simulink model "Ex1s"  (R2025a)
settings: Solver=VariableStepAuto  StartTime=0.0  StopTime=10.0  RelTol=1e-3

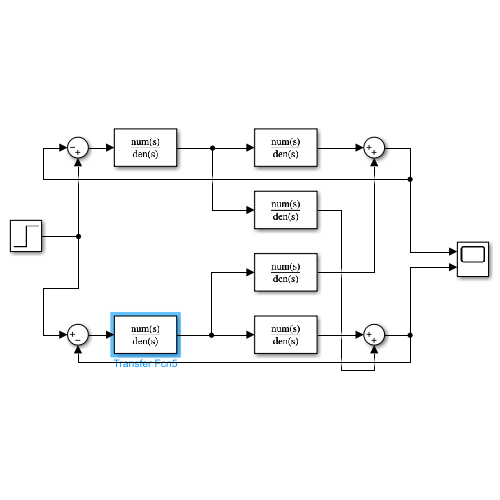
[thumbnail: Simulink's stored preview of the top-level diagram]
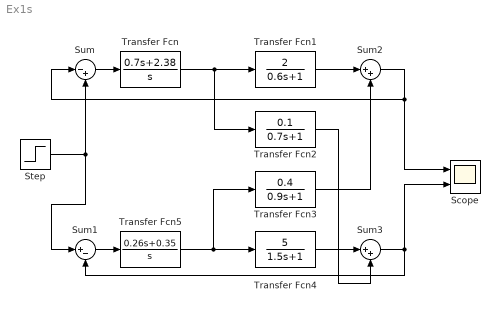
== system Ex1s ==
  Scope : Scope  NumInputPorts=2
      settings: ActiveDisplayYMinimum=-0.092364806170674857  ActiveDisplayYMaximum=0.83128325553607385
  Step : Step  SampleTime=0
  Sum : Sum  Inputs=|-+
  Sum1 : Sum  Inputs=|+-
  Sum2 : Sum  Inputs=|++
  Sum3 : Sum  Inputs=|++
  Transfer Fcn : TransferFcn  Numerator=[0.7 2.38]  Denominator=[1 0]
  Transfer Fcn1 : TransferFcn  Numerator=2  Denominator=[0.6 1]
  Transfer Fcn2 : TransferFcn  Numerator=0.1  Denominator=[0.7 1]
  Transfer Fcn3 : TransferFcn  Numerator=0.4  Denominator=[0.9 1]
  Transfer Fcn4 : TransferFcn  Numerator=[5]  Denominator=[1.5 1]
  Transfer Fcn5 : TransferFcn  Numerator=[0.26 0.35]  Denominator=[1 0]
  wires:
  Step/1 -> Sum/2, Sum1/1
  Transfer Fcn5/1 -> Transfer Fcn3/1, Transfer Fcn4/1
  Transfer Fcn/1 -> Transfer Fcn2/1, Transfer Fcn1/1
  Sum/1 -> Transfer Fcn/1
  Sum1/1 -> Transfer Fcn5/1
  Transfer Fcn1/1 -> Sum2/1
  Transfer Fcn4/1 -> Sum3/1
  Transfer Fcn2/1 -> Sum3/2
  Transfer Fcn3/1 -> Sum2/2
  Sum3/1 -> Scope/2, Sum1/2
  Sum2/1 -> Scope/1, Sum/1
